simulink model "SimulinkModel"  (R2022b)
settings: Solver=FixedStepAuto  StartTime=0.0  StopTime=10.0  FixedStep=1e-06  RelTol=1e-3
settings Model: DataDictionary=BusSystem.sldd  Creator=cao2851  LastModifiedBy=cao2851

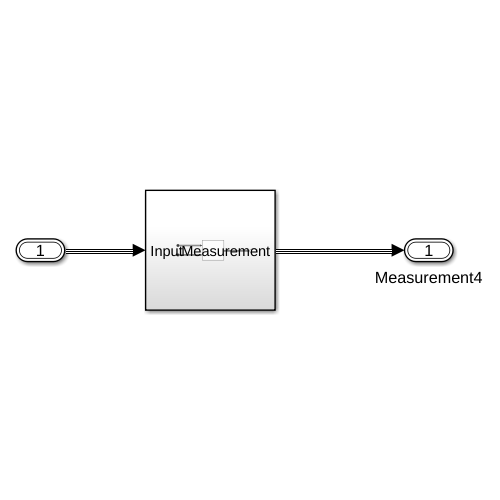
[thumbnail: Simulink's stored preview of the top-level diagram]
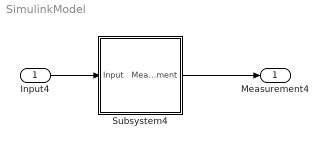
== system SimulinkModel ==
  Input4 : Inport  OutDataTypeStr=Bus: bus7
  Subsystem4 : Subsystem
  Measurement4 : Outport  OutDataTypeStr=Bus: slBus1
  wires:
  Subsystem4/1(Measurement) -> Measurement4/1
  Input4/1 -> Subsystem4/1(Input)

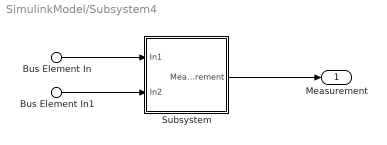
== system SimulinkModel/Subsystem4 ==
  Bus Element In : Inport  PortName=Input  Element=signal1
  Bus Element In1 : Inport  PortName=Input  Element=Signal2
  Subsystem : Subsystem
  Measurement : Outport
  wires:
  Subsystem/1(Measurement) -> Measurement/1
  Bus Element In1/1 -> Subsystem/2(In2)
  Bus Element In/1 -> Subsystem/1(In1)

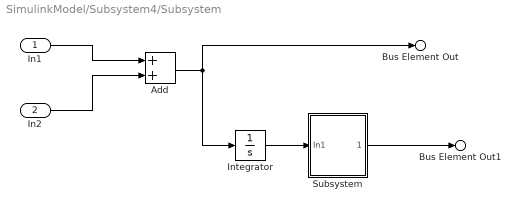
== system SimulinkModel/Subsystem4/Subsystem ==
  In1 : Inport
  In2 : Inport  Port=2
  Add : Sum
  Integrator : Integrator
  Subsystem : Subsystem
  Bus Element Out : Outport  PortName=Measurement  Element=add
  Bus Element Out1 : Outport  PortName=Measurement  Element=integrator
  wires:
  Subsystem/1(Measurement) -> Bus Element Out1/1
  Integrator/1 -> Subsystem/1(In1)
  Add/1 -> Bus Element Out/1, Integrator/1
  In2/1 -> Add/2
  In1/1 -> Add/1

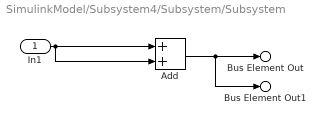
== system SimulinkModel/Subsystem4/Subsystem/Subsystem ==
  In1 : Inport
  Add : Sum
  Bus Element Out : Outport  PortName=Measurement  Element=signal1
  Bus Element Out1 : Outport  PortName=Measurement  Element=signal2
  wires:
  Add/1 -> Bus Element Out/1, Bus Element Out1/1
  In1/1 -> Add/1, Add/2
